simulink model "example_P_1"  (R2018a)
settings: Solver=VariableStepAuto  StartTime=0.0  StopTime=10.0  RelTol=1e-6
settings Model: Creator=gbecerra  LastModifiedBy=gbecerra

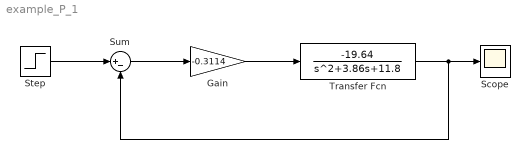
== system example_P_1 ==
  Gain : Gain  Gain=-0.3114
  Scope : Scope
  Step : Step  Time=0  SampleTime=0
  Sum : Sum  Inputs=|+-
  Transfer Fcn : TransferFcn  Numerator=[-19.64]  Denominator=[1 3.86 11.8]
  wires:
  Gain/1 -> Transfer Fcn/1
  Step/1 -> Sum/1
  Sum/1 -> Gain/1
  Transfer Fcn/1 -> Scope/1, Sum/2
